simulink model "BandwidthSelector"  (R2019a)
settings: Solver=VariableStepAuto  StartTime=0.0  StopTime=inf  RelTol=1e-3
InitFcn:
  | bandwidthselector_setup;
values from neighbouring files (symbols this model uses):
  f = 256e6    (= 256000000)    [bandwidthselector_setup.m]
undefined symbols (not defined in the file or in its folder): AXI4, designMultirateFIR, Lite, xlfda_numerator
libraries: xbsIndex_r4 x43, dspmlti4 x6, dspswit3 x4, dspsigops x2
(part 1 of 2)
settings Model: Creator=rgb11127  LastModifiedBy=david
settings DataIOCC: ReturnWorkspaceOutputs=off
settings DebuggingCC: PregeneratedLibrarySubsystemCodeDiagnostic=none  ArithmeticOperatorsInVariantConditions=warning
settings SFSimCC: SimUseLocalCustomCode=off
settings RTWCC: RTWUseLocalCustomCode=off

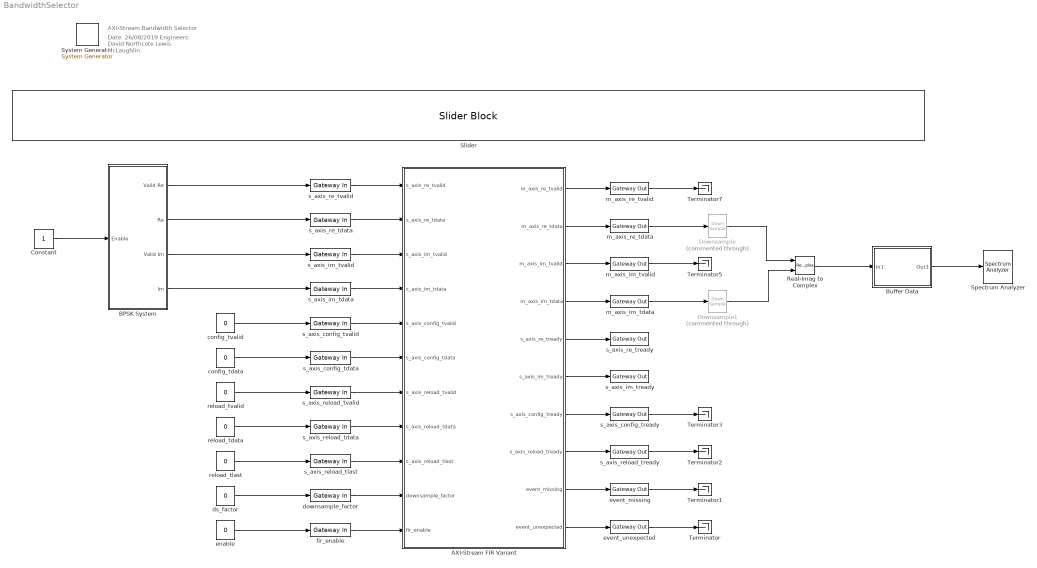
== system BandwidthSelector ==
  note: Date: 26/08/2019
      | Engineers: David Northcote
      | Lewis McLaughlin
  note: AXI-Stream Bandwidth Selector
  " System Generator" : xbsIndex_r4/ System Generator  Tag=genX  xilinxfamily=zynquplusRFSOC  part=xczu28dr  speed=-2-e  package=ffvg1517  synthesis_tool=Vivado  clock_wrapper=Clock Enables  directory=./netlist  proj_type=Vivado  Synth_file=Vivado Synthesis Defaults  Impl_file=Vivado Implementation Defaults  testbench=off  simulink_period=1/f  sysclk_period=(1/f)*1e9  dcm_input_clock_period=10  incr_netlist=off  trim_vbits=Everywhere in SubSystem  dbl_ovrd=According to Block Masks  core_generation=According to Block Masks  run_coregen=off  deprecated_control=off  eval_field=0  block_type=sysgen
  AXI-Stream FIR Variant : Subsystem  AncestorBlock=lib_fir/AXI-Stream FIR Variant  VariantControlMode=Label  Variant=on  VariantControl=Variant1  LabelModeActiveChoice=Variant
  BPSK System : Subsystem
  Buffer Data : Subsystem
  Constant : Constant  SampleTime=-1
  Downsample : DownSample  Commented=through  N=1  RateOptions=Allow multirate processing
  Downsample1 : DownSample  Commented=through  N=1  RateOptions=Allow multirate processing
  Real-Imag to Complex : RealImagToComplex
  Slider : SliderBlock  ScaleMax=128000000  TickInterval=4000000
  Spectrum Analyzer : SpectrumAnalyzer
  Terminator{,1..3,5,7} (6 alike) : Terminator
  config_tdata : Constant  Value=0  OutDataTypeStr=fixdt(0,8,0)  SampleTime=1/f
  config_tvalid : Constant  Value=0  OutDataTypeStr=boolean  SampleTime=1/f
  downsample_factor : xbsIndex_r4/Gateway In  gui_display_data_type=Fixed-point  arith_type=Unsigned  n_bits=32  bin_pt=0  preci_type=Single  exp_width=8  frac_width=24  rows=1  columns=1  quantization=Truncate  overflow=Wrap  period=1/f  UseAsADC=off  ADCChannel='1'  interface=AXI4-Lite  automatic_assignment=on  address_offset=hex2dec('00')  intf_name=''  intf_description=''  default_value=1  timing_constraint=None  locs_specified=off  LOCs={}  io_standard={}  inherit_from_input=off  hdl_port=on  dbl_ovrd=off  block_type=gatewayin
  ds_factor : Constant  Value=0  OutDataTypeStr=uint16  SampleTime=1/f
  enable : Constant  Value=0  OutDataTypeStr=uint32  SampleTime=1/f
  event_missing : xbsIndex_r4/Gateway Out  inherit_from_input=on  hdl_port=on  rows=1  columns=1  UseAsDAC=off  DACChannel='1'  interface=AXI4-Lite  automatic_assignment=on  address_offset=hex2dec('00')  intf_name=''  intf_description=''  timing_constraint=None  locs_specified=off  LOCs={}  io_standard={}  block_type=gatewayout
  event_unexpected : xbsIndex_r4/Gateway Out  inherit_from_input=on  hdl_port=on  rows=1  columns=1  UseAsDAC=off  DACChannel='1'  interface=AXI4-Lite  automatic_assignment=on  address_offset=hex2dec('00')  intf_name=''  intf_description=''  timing_constraint=None  locs_specified=off  LOCs={}  io_standard={}  block_type=gatewayout
  fir_enable : xbsIndex_r4/Gateway In  gui_display_data_type=Fixed-point  arith_type=Unsigned  n_bits=8  bin_pt=0  preci_type=Single  exp_width=8  frac_width=24  rows=1  columns=1  quantization=Truncate  overflow=Saturate  period=1/f  UseAsADC=off  ADCChannel='1'  interface=AXI4-Lite  automatic_assignment=on  address_offset=hex2dec('00')  intf_name=''  intf_description=''  default_value=1  timing_constraint=None  locs_specified=off  LOCs={}  io_standard={}  inherit_from_input=off  hdl_port=on  dbl_ovrd=off  block_type=gatewayin
  m_axis_im_tdata : xbsIndex_r4/Gateway Out  inherit_from_input=on  hdl_port=on  rows=1  columns=1  UseAsDAC=off  DACChannel='1'  interface=None  automatic_assignment=on  address_offset=hex2dec('00')  intf_name=''  intf_description=''  timing_constraint=None  locs_specified=off  LOCs={}  io_standard={}  block_type=gatewayout
  m_axis_im_tvalid : xbsIndex_r4/Gateway Out  inherit_from_input=on  hdl_port=on  rows=1  columns=1  UseAsDAC=off  DACChannel='1'  interface=None  automatic_assignment=on  address_offset=hex2dec('00')  intf_name=''  intf_description=''  timing_constraint=None  locs_specified=off  LOCs={}  io_standard={}  block_type=gatewayout
  m_axis_re_tdata : xbsIndex_r4/Gateway Out  inherit_from_input=on  hdl_port=on  rows=1  columns=1  UseAsDAC=off  DACChannel='1'  interface=None  automatic_assignment=on  address_offset=hex2dec('00')  intf_name=''  intf_description=''  timing_constraint=None  locs_specified=off  LOCs={}  io_standard={}  block_type=gatewayout
  m_axis_re_tvalid : xbsIndex_r4/Gateway Out  inherit_from_input=on  hdl_port=on  rows=1  columns=1  UseAsDAC=off  DACChannel='1'  interface=None  automatic_assignment=on  address_offset=hex2dec('00')  intf_name=''  intf_description=''  timing_constraint=None  locs_specified=off  LOCs={}  io_standard={}  block_type=gatewayout
  reload_tdata : Constant  Value=0  OutDataTypeStr=fixdt(0,12,0)  SampleTime=1/f
  reload_tlast : Constant  Value=0  OutDataTypeStr=boolean  SampleTime=1/f
  reload_tvalid : Constant  Value=0  OutDataTypeStr=boolean  SampleTime=1/f
  s_axis_config_tdata : xbsIndex_r4/Gateway In  gui_display_data_type=Fixed-point  arith_type=Unsigned  n_bits=8  bin_pt=0  preci_type=Single  exp_width=8  frac_width=24  rows=1  columns=1  quantization="Round  (unbiased: +/- Inf)"  overflow=Saturate  period=1/f  UseAsADC=off  ADCChannel='1'  interface=None  automatic_assignment=on  address_offset=hex2dec('00')  intf_name=''  intf_description=''  default_value=0  timing_constraint=None  locs_specified=off  LOCs={}  io_standard={}  inherit_from_input=off  hdl_port=on  dbl_ovrd=off  block_type=gatewayin
  s_axis_config_tready : xbsIndex_r4/Gateway Out  inherit_from_input=on  hdl_port=on  rows=1  columns=1  UseAsDAC=off  DACChannel='1'  interface=None  automatic_assignment=on  address_offset=hex2dec('00')  intf_name=''  intf_description=''  timing_constraint=None  locs_specified=off  LOCs={}  io_standard={}  block_type=gatewayout
  s_axis_config_tvalid : xbsIndex_r4/Gateway In  gui_display_data_type=Boolean  arith_type=Boolean  n_bits=16  bin_pt=14  preci_type=Single  exp_width=8  frac_width=24  rows=1  columns=1  quantization="Round  (unbiased: +/- Inf)"  overflow=Saturate  period=1/f  UseAsADC=off  ADCChannel='1'  interface=None  automatic_assignment=on  address_offset=hex2dec('00')  intf_name=''  intf_description=''  default_value=0  timing_constraint=None  locs_specified=off  LOCs={}  io_standard={}  inherit_from_input=off  hdl_port=on  dbl_ovrd=off  block_type=gatewayin
  s_axis_im_tdata : xbsIndex_r4/Gateway In  gui_display_data_type=Fixed-point  arith_type="Signed  (2's comp)"  n_bits=16  bin_pt=15  preci_type=Single  exp_width=8  frac_width=24  rows=1  columns=1  quantization="Round  (unbiased: +/- Inf)"  overflow=Saturate  period=1/f  UseAsADC=off  ADCChannel='1'  interface=None  automatic_assignment=on  address_offset=hex2dec('00')  intf_name=''  intf_description=''  default_value=0  timing_constraint=None  locs_specified=off  LOCs={}  io_standard={}  inherit_from_input=off  hdl_port=on  dbl_ovrd=off  block_type=gatewayin
  s_axis_im_tready : xbsIndex_r4/Gateway Out  inherit_from_input=on  hdl_port=on  rows=1  columns=1  UseAsDAC=off  DACChannel='1'  interface=None  automatic_assignment=on  address_offset=hex2dec('00')  intf_name=''  intf_description=''  timing_constraint=None  locs_specified=off  LOCs={}  io_standard={}  block_type=gatewayout
  s_axis_im_tvalid : xbsIndex_r4/Gateway In  gui_display_data_type=Boolean  arith_type=Boolean  n_bits=16  bin_pt=14  preci_type=Single  exp_width=8  frac_width=24  rows=1  columns=1  quantization="Round  (unbiased: +/- Inf)"  overflow=Saturate  period=1/f  UseAsADC=off  ADCChannel='1'  interface=None  automatic_assignment=on  address_offset=hex2dec('00')  intf_name=''  intf_description=''  default_value=0  timing_constraint=None  locs_specified=off  LOCs={}  io_standard={}  inherit_from_input=off  hdl_port=on  dbl_ovrd=off  block_type=gatewayin
  s_axis_re_tdata : xbsIndex_r4/Gateway In  gui_display_data_type=Fixed-point  arith_type="Signed  (2's comp)"  n_bits=16  bin_pt=15  preci_type=Single  exp_width=8  frac_width=24  rows=1  columns=1  quantization="Round  (unbiased: +/- Inf)"  overflow=Saturate  period=1/f  UseAsADC=off  ADCChannel='1'  interface=None  automatic_assignment=on  address_offset=hex2dec('00')  intf_name=''  intf_description=''  default_value=0  timing_constraint=None  locs_specified=off  LOCs={}  io_standard={}  inherit_from_input=off  hdl_port=on  dbl_ovrd=off  block_type=gatewayin
  s_axis_re_tready : xbsIndex_r4/Gateway Out  inherit_from_input=on  hdl_port=on  rows=1  columns=1  UseAsDAC=off  DACChannel='1'  interface=None  automatic_assignment=on  address_offset=hex2dec('00')  intf_name=''  intf_description=''  timing_constraint=None  locs_specified=off  LOCs={}  io_standard={}  block_type=gatewayout
  s_axis_re_tvalid : xbsIndex_r4/Gateway In  gui_display_data_type=Boolean  arith_type=Boolean  n_bits=16  bin_pt=14  preci_type=Single  exp_width=8  frac_width=24  rows=1  columns=1  quantization="Round  (unbiased: +/- Inf)"  overflow=Saturate  period=1/f  UseAsADC=off  ADCChannel='1'  interface=None  automatic_assignment=on  address_offset=hex2dec('00')  intf_name=''  intf_description=''  default_value=0  timing_constraint=None  locs_specified=off  LOCs={}  io_standard={}  inherit_from_input=off  hdl_port=on  dbl_ovrd=off  block_type=gatewayin
  s_axis_reload_tdata : xbsIndex_r4/Gateway In  gui_display_data_type=Fixed-point  arith_type=Unsigned  n_bits=16  bin_pt=0  preci_type=Single  exp_width=8  frac_width=24  rows=1  columns=1  quantization="Round  (unbiased: +/- Inf)"  overflow=Saturate  period=1/f  UseAsADC=off  ADCChannel='1'  interface=None  automatic_assignment=on  address_offset=hex2dec('00')  intf_name=''  intf_description=''  default_value=0  timing_constraint=None  locs_specified=off  LOCs={}  io_standard={}  inherit_from_input=off  hdl_port=on  dbl_ovrd=off  block_type=gatewayin
  s_axis_reload_tlast : xbsIndex_r4/Gateway In  gui_display_data_type=Boolean  arith_type=Boolean  n_bits=16  bin_pt=14  preci_type=Single  exp_width=8  frac_width=24  rows=1  columns=1  quantization="Round  (unbiased: +/- Inf)"  overflow=Saturate  period=1/f  UseAsADC=off  ADCChannel='1'  interface=None  automatic_assignment=on  address_offset=hex2dec('00')  intf_name=''  intf_description=''  default_value=0  timing_constraint=None  locs_specified=off  LOCs={}  io_standard={}  inherit_from_input=off  hdl_port=on  dbl_ovrd=off  block_type=gatewayin
  s_axis_reload_tready : xbsIndex_r4/Gateway Out  inherit_from_input=on  hdl_port=on  rows=1  columns=1  UseAsDAC=off  DACChannel='1'  interface=None  automatic_assignment=on  address_offset=hex2dec('00')  intf_name=''  intf_description=''  timing_constraint=None  locs_specified=off  LOCs={}  io_standard={}  block_type=gatewayout
  s_axis_reload_tvalid : xbsIndex_r4/Gateway In  gui_display_data_type=Boolean  arith_type=Boolean  n_bits=16  bin_pt=14  preci_type=Single  exp_width=8  frac_width=24  rows=1  columns=1  quantization="Round  (unbiased: +/- Inf)"  overflow=Saturate  period=1/f  UseAsADC=off  ADCChannel='1'  interface=None  automatic_assignment=on  address_offset=hex2dec('00')  intf_name=''  intf_description=''  default_value=0  timing_constraint=None  locs_specified=off  LOCs={}  io_standard={}  inherit_from_input=off  hdl_port=on  dbl_ovrd=off  block_type=gatewayin
  wires:
  reload_tlast/1 -> s_axis_reload_tlast/1
  reload_tdata/1 -> s_axis_reload_tdata/1
  config_tdata/1 -> s_axis_config_tdata/1
  reload_tvalid/1 -> s_axis_reload_tvalid/1
  config_tvalid/1 -> s_axis_config_tvalid/1
  AXI-Stream FIR Variant/5(s_axis_re_tready) -> s_axis_re_tready/1
  AXI-Stream FIR Variant/6(s_axis_im_tready) -> s_axis_im_tready/1
  AXI-Stream FIR Variant/10(event_unexpected) -> event_unexpected/1
  AXI-Stream FIR Variant/9(event_missing) -> event_missing/1
  AXI-Stream FIR Variant/8(" s_axis_reload_tready") -> s_axis_reload_tready/1
  AXI-Stream FIR Variant/7(" s_axis_config_tready") -> s_axis_config_tready/1
  AXI-Stream FIR Variant/4(" m_axis_im_tdata") -> m_axis_im_tdata/1
  AXI-Stream FIR Variant/3(" m_axis_im_tvalid") -> m_axis_im_tvalid/1
  AXI-Stream FIR Variant/2(" m_axis_re_tdata") -> m_axis_re_tdata/1
  AXI-Stream FIR Variant/1(" m_axis_re_tvalid") -> m_axis_re_tvalid/1
  s_axis_re_tvalid/1 -> AXI-Stream FIR Variant/1("s_axis_re_tvalid ")
  s_axis_im_tvalid/1 -> AXI-Stream FIR Variant/3(s_axis_im_tvalid)
  s_axis_re_tdata/1 -> AXI-Stream FIR Variant/2(s_axis_re_tdata)
  s_axis_im_tdata/1 -> AXI-Stream FIR Variant/4(s_axis_im_tdata)
  s_axis_config_tvalid/1 -> AXI-Stream FIR Variant/5(s_axis_config_tvalid)
  s_axis_reload_tvalid/1 -> AXI-Stream FIR Variant/7(s_axis_reload_tvalid)
  s_axis_reload_tlast/1 -> AXI-Stream FIR Variant/9(s_axis_reload_tlast)
  s_axis_config_tdata/1 -> AXI-Stream FIR Variant/6(s_axis_config_tdata)
  s_axis_reload_tdata/1 -> AXI-Stream FIR Variant/8(s_axis_reload_tdata)
  m_axis_re_tvalid/1 -> Terminator7/1
  m_axis_im_tvalid/1 -> Terminator5/1
  s_axis_config_tready/1 -> Terminator3/1
  s_axis_reload_tready/1 -> Terminator2/1
  event_missing/1 -> Terminator1/1
  event_unexpected/1 -> Terminator/1
  Constant/1 -> BPSK System/1(Enable)
  downsample_factor/1 -> AXI-Stream FIR Variant/10(downsample_factor)
  ds_factor/1 -> downsample_factor/1
  enable/1 -> fir_enable/1
  fir_enable/1 -> AXI-Stream FIR Variant/11(fir_enable)
  Downsample/1 -> Real-Imag to Complex/1
  Downsample1/1 -> Real-Imag to Complex/2
  Real-Imag to Complex/1 -> Buffer Data/1(In1)
  Buffer Data/1(Out1) -> Spectrum Analyzer/1
  m_axis_im_tdata/1 -> Downsample1/1
  m_axis_re_tdata/1 -> Downsample/1
  BPSK System/2(Re) -> s_axis_re_tdata/1
  BPSK System/1(Valid Re) -> s_axis_re_tvalid/1
  BPSK System/3(Valid Im) -> s_axis_im_tvalid/1
  BPSK System/4(Im) -> s_axis_im_tdata/1

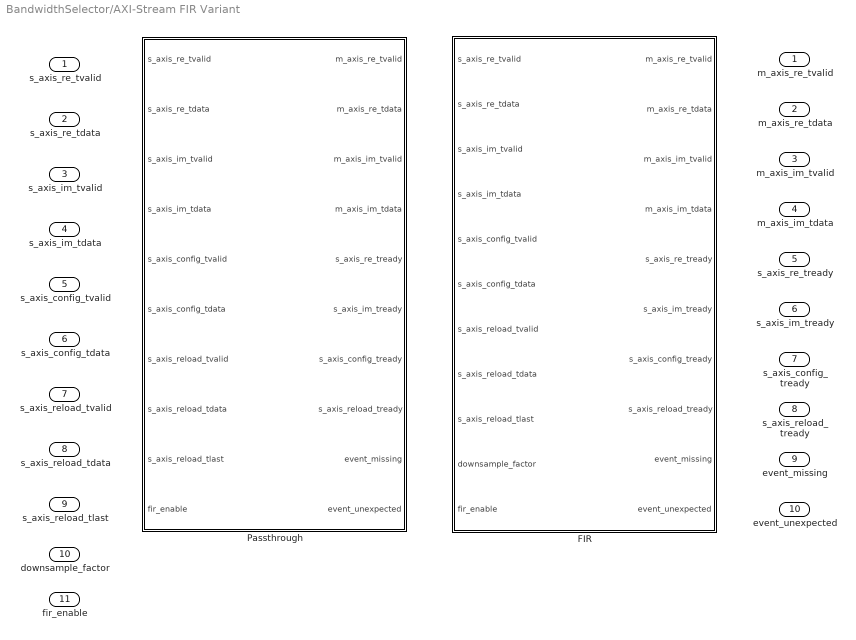
== system BandwidthSelector/AXI-Stream FIR Variant ==
  "s_axis_re_tvalid " : Inport
  s_axis_re_tdata : Inport  Port=2
  s_axis_im_tvalid : Inport  Port=3
  s_axis_im_tdata : Inport  Port=4
  s_axis_config_tvalid : Inport  Port=5
  s_axis_config_tdata : Inport  Port=6
  s_axis_reload_tvalid : Inport  Port=7
  s_axis_reload_tdata : Inport  Port=8
  s_axis_reload_tlast : Inport  Port=9
  downsample_factor : Inport  Port=10
  fir_enable : Inport  Port=11
  FIR : Subsystem  VariantControl=Variant
  Passthrough : Subsystem  VariantControl=Variant1
  " m_axis_re_tvalid" : Outport
  " m_axis_re_tdata" : Outport  Port=2
  " m_axis_im_tvalid" : Outport  Port=3
  " m_axis_im_tdata" : Outport  Port=4
  s_axis_re_tready : Outport  Port=5
  s_axis_im_tready : Outport  Port=6
  " s_axis_config_tready" : Outport  Port=7
  " s_axis_reload_tready" : Outport  Port=8
  event_missing : Outport  Port=9
  event_unexpected : Outport  Port=10

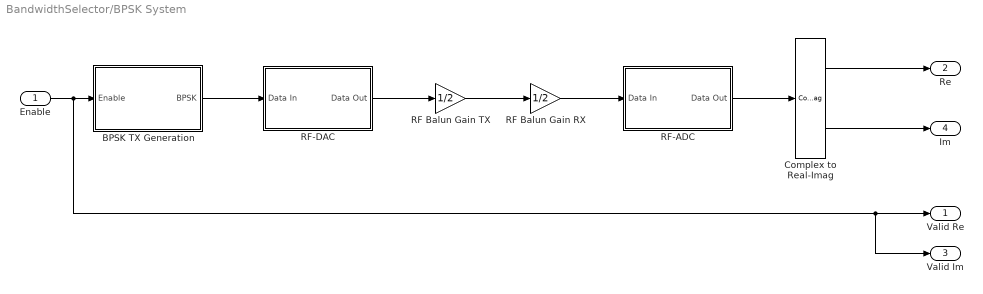
== system BandwidthSelector/BPSK System ==
  Enable : Inport
  BPSK TX Generation : Subsystem
  Complex to Real-Imag : ComplexToRealImag
  RF Balun Gain RX : Gain  Gain=1/2
  RF Balun Gain TX : Gain  Gain=1/2
  RF-ADC : Subsystem  mask{fs_ghz=2.048, decim=8x, ssr=1, mode=Fine, fc=0.064, fph=0, fcoarse=fs/4}
      mask prompts: fs_ghz "Sample Rate (GHz):"; decim "Interpolation Mode:"; ssr "Samples per AXI4-Stream Cycle:"; mode "Mixer Type:"; fc "NCO Frequency (GHz):"; fph "NCO Phase (Rads):"; fcoarse "Frequency:"
      mask init:
      | % Obtain the sample rate in Hz
      | fs = str2double(get_param(gcb, 'fs_ghz'))*1e9;
      | 
      | % Set the mode of the RF-DAC interpolation filter
      | switch get_param(gcb, 'decim')
      |     case '1x'
      |         D = 1;
      |     case '2x'
      |         D = 2;
      |     case '4x'
      |         D = 4;
      |     case '8x'
      |         D = 8;
      |     otherwise
      |         D = 1;
      | end
      | 
      | % Get the AXI-Stream clock for display to user
      | axi_clk = (fs/(str2double(get_param(gcb, 'ssr'))*D))*1e-6;
      | 
      | % Get the block mask object to manipulate settings
      | mo = get_param(gcb, 'MaskObject');
      | 
      | % Update text to display the required AXI-Stream clock
      | tc = mo.getDialogControl('axi_text');
      | tc.Prompt = ['      Required AXI-Stream Clock: ', num2str(axi_clk), ' MHz'];
      | 
      | % Set the RF-DAC Mixer mode
      | switch get_param(gcb, 'mode')
      |     case 'Bypass'
      |         m = 0;
      |     case 'Coarse'
      |         m = 1;
      |     case 'Fine'
      |         m = 2;
      |     otherwise
      |         m = 0;
      | end
      | 
      | % Set the RF-DAC Coarse Mixer mode
      | switch get_param(gcb, 'fcoarse')
      |     case 'fs/2'
      |         mc = 0;
      |     case 'fs/4'
      |         mc = 1;
      |     case '-fs/4'
      |         mc = 2;
      |     otherwise
      |         mc = 0;
      | end
      | 
      | % Set other blocks
      | set_param([gcb, '/Decimation Filter'], 'decim', get_param(gcb, 'decim'));
      mask Callback fs_ghz:
      | % Obtain the sample rate in Hz
      | fs = str2double(get_param(gcb, 'fs_ghz'))*1e9;
      | 
      | % Set the mode of the RF-DAC interpolation filter
      | switch get_param(gcb, 'decim')
      |     case '1x'
      |         D = 1;
      |     case '2x'
      |         D = 2;
      |     case '4x'
      |         D = 4;
      |     case '8x'
      |         D = 8;
      |     otherwise
      |         D = 1;
      | end
      | 
      | % Get the AXI-Stream clock for display to user
      | axi_clk = (fs/(str2double(get_param(gcb, 'ssr'))*D))*1e-6;
      | 
      | % Get the block mask object to manipulate settings
      | mo = get_param(gcb, 'MaskObject');
      | 
      | % Update text to display the required AXI-Stream clock
      | tc = mo.getDialogControl('axi_text');
      | tc.Prompt = ['      Required AXI-Stream Clock: ', num2str(axi_clk), ' MHz'];
      mask TypeOptions decim: 1x | 2x | 4x | 8x
      mask Callback decim:
      | % Obtain the sample rate in Hz
      | fs = str2double(get_param(gcb, 'fs_ghz'))*1e9;
      | 
      | % Set the mode of the RF-DAC interpolation filter
      | switch get_param(gcb, 'decim')
      |     case '1x'
      |         D = 1;
      |     case '2x'
      |         D = 2;
      |     case '4x'
      |         D = 4;
      |     case '8x'
      |         D = 8;
      |     otherwise
      |         D = 1;
      | end
      | 
      | % Get the AXI-Stream clock for display to user
      | axi_clk = (fs/(str2double(get_param(gcb, 'ssr'))*D))*1e-6;
      | 
      | % Get the block mask object to manipulate settings
      | mo = get_param(gcb, 'MaskObject');
      | 
      | % Update text to display the required AXI-Stream clock
      | tc = mo.getDialogControl('axi_text');
      | tc.Prompt = ['      Required AXI-Stream Clock: ', num2str(axi_clk), ' MHz'];
      mask TypeOptions ssr: 1 | 2 | 3 | 4 | 5 | 6 | 7 | 8 | 9 | 10 | 11 | 12 | 13 | 14 | 15 | 16
      mask Callback ssr:
      | % Obtain the sample rate in Hz
      | fs = str2double(get_param(gcb, 'fs_ghz'))*1e9;
      | 
      | % Set the mode of the RF-DAC interpolation filter
      | switch get_param(gcb, 'decim')
      |     case '1x'
      |         D = 1;
      |     case '2x'
      |         D = 2;
      |     case '4x'
      |         D = 4;
      |     case '8x'
      |         D = 8;
      |     otherwise
      |         D = 1;
      | end
      | 
      | % Get the AXI-Stream clock for display to user
      | axi_clk = (fs/(str2double(get_param(gcb, 'ssr'))*D))*1e-6;
      | 
      | % Get the block mask object to manipulate settings
      | mo = get_param(gcb, 'MaskObject');
      | 
      | % Update text to display the required AXI-Stream clock
      | tc = mo.getDialogControl('axi_text');
      | tc.Prompt = ['      Required AXI-Stream Clock: ', num2str(axi_clk), ' MHz'];
      mask TypeOptions mode: Coarse | Fine
      mask Callback mode:
      | % Get the block mask object to manipulate settings
      | mo = get_param(gcb, 'MaskObject');
      | 
      | % Hide group depending on Mixer mode choice
      | switch get_param(gcb, 'mode')
      |     case 'Bypass'
      |         mo.getDialogControl('coarse_group').Visible='off';
      |         mo.getDialogControl('mixer_group').Visible='off';
      |     case 'Coarse'
      |         mo.getDialogControl('coarse_group').Visible='on';
      |         mo.getDialogControl('mixer_group').Visible='off';
      |     case 'Fine'
      |         mo.getDialogControl('coarse_group').Visible='off';
      |         mo.getDialogControl('mixer_group').Visible='on';
      |     otherwise
      |         mo.getDialogControl('coarse_group').Visible='off';
      |         mo.getDialogControl('mixer_group').Visible='off';
      | end
      mask TypeOptions fcoarse: fs/2 | fs/4 | -fs/4
      mask DialogControl DescGroupVar Prompt: RF-DAC
      mask DialogControl DescTextVar Prompt: This block simulates one RF-ADC channel.
      mask DialogControl main_group Prompt: Data Settings
      mask DialogControl axi_text Prompt: Required AXI-Stream Clock: 256 MHz
      mask DialogControl Container5 Prompt: Mixer Settings
  RF-DAC : Subsystem  mask{fs_ghz=2.048, interp=8x, ssr=1, mode=Fine, fc=0.032, fph=0, fcoarse=fs/4}
      mask prompts: fs_ghz "Sample Rate (GHz):"; interp "Interpolation Mode:"; ssr "Samples per AXI4-Stream Cycle:"; mode "Mixer Type:"; fc "NCO Frequency (GHz):"; fph "NCO Phase (Rads):"; fcoarse "Frequency:"
      mask init:
      | % Obtain the sample rate in Hz
      | fs = str2double(get_param(gcb, 'fs_ghz'))*1e9;
      | 
      | % Set the mode of the RF-DAC interpolation filter
      | switch get_param(gcb, 'interp')
      |     case '1x'
      |         L = 1;
      |     case '2x'
      |         L = 2;
      |     case '4x'
      |         L = 4;
      |     case '8x'
      |         L = 8;
      |     otherwise
      |         L = 1;
      | end
      | 
      | % Get the AXI-Stream clock for display to user
      | axi_clk = (fs/(str2double(get_param(gcb, 'ssr'))*L))*1e-6;
      | 
      | % Get the block mask object to manipulate settings
      | mo = get_param(gcb, 'MaskObject');
      | 
      | % Update text to display the required AXI-Stream clock
      | tc = mo.getDialogControl('axi_text');
      | tc.Prompt = ['      Required AXI-Stream Clock: ', num2str(axi_clk), ' MHz'];
      | 
      | % Set the RF-DAC Mixer mode
      | switch get_param(gcb, 'mode')
      |     case 'Bypass'
      |         m = 0;
      |     case 'Coarse'
      |         m = 1;
      |     case 'Fine'
      |         m = 2;
      |     otherwise
      |         m = 0;
      | end
      | 
      | % Set the RF-DAC Coarse Mixer mode
      | switch get_param(gcb, 'fcoarse')
      |     case 'fs/2'
      |         mc = 0;
      |     case 'fs/4'
      |         mc = 1;
      |     case '-fs/4'
      |         mc = 2;
      |     otherwise
      |         mc = 0;
      | end
      | 
      | % Set other blocks
      | set_param([gcb, '/Interpolation Filter'], 'interp', get_param(gcb, 'interp'));
      mask Callback fs_ghz:
      | % Obtain the sample rate in Hz
      | fs = str2double(get_param(gcb, 'fs_ghz'))*1e9;
      | 
      | % Set the mode of the RF-DAC interpolation filter
      | switch get_param(gcb, 'interp')
      |     case '1x'
      |         L = 1;
      |     case '2x'
      |         L = 2;
      |     case '4x'
      |         L = 4;
      |     case '8x'
      |         L = 8;
      |     otherwise
      |         L = 1;
      | end
      | 
      | % Get the AXI-Stream clock for display to user
      | axi_clk = (fs/(str2double(get_param(gcb, 'ssr'))*L))*1e-6;
      | 
      | % Get the block mask object to manipulate settings
      | mo = get_param(gcb, 'MaskObject');
      | 
      | % Update text to display the required AXI-Stream clock
      | tc = mo.getDialogControl('axi_text');
      | tc.Prompt = ['      Required AXI-Stream Clock: ', num2str(axi_clk), ' MHz'];
      mask TypeOptions interp: 1x | 2x | 4x | 8x
      mask Callback interp:
      | % Obtain the sample rate in Hz
      | fs = str2double(get_param(gcb, 'fs_ghz'))*1e9;
      | 
      | % Set the mode of the RF-DAC interpolation filter
      | switch get_param(gcb, 'interp')
      |     case '1x'
      |         L = 1;
      |     case '2x'
      |         L = 2;
      |     case '4x'
      |         L = 4;
      |     case '8x'
      |         L = 8;
      |     otherwise
      |         L = 1;
      | end
      | 
      | % Get the AXI-Stream clock for display to user
      | axi_clk = (fs/(str2double(get_param(gcb, 'ssr'))*L))*1e-6;
      | 
      | % Get the block mask object to manipulate settings
      | mo = get_param(gcb, 'MaskObject');
      | 
      | % Update text to display the required AXI-Stream clock
      | tc = mo.getDialogControl('axi_text');
      | tc.Prompt = ['      Required AXI-Stream Clock: ', num2str(axi_clk), ' MHz'];
      mask TypeOptions ssr: 1 | 2 | 3 | 4 | 5 | 6 | 7 | 8 | 9 | 10 | 11 | 12 | 13 | 14 | 15 | 16
      mask Callback ssr:
      | % Obtain the sample rate in Hz
      | fs = str2double(get_param(gcb, 'fs_ghz'))*1e9;
      | 
      | % Set the mode of the RF-DAC interpolation filter
      | switch get_param(gcb, 'interp')
      |     case '1x'
      |         L = 1;
      |     case '2x'
      |         L = 2;
      |     case '4x'
      |         L = 4;
      |     case '8x'
      |         L = 8;
      |     otherwise
      |         L = 1;
      | end
      | 
      | % Get the AXI-Stream clock for display to user
      | axi_clk = (fs/(str2double(get_param(gcb, 'ssr'))*L))*1e-6;
      | 
      | % Get the block mask object to manipulate settings
      | mo = get_param(gcb, 'MaskObject');
      | 
      | % Update text to display the required AXI-Stream clock
      | tc = mo.getDialogControl('axi_text');
      | tc.Prompt = ['      Required AXI-Stream Clock: ', num2str(axi_clk), ' MHz'];
      mask TypeOptions mode: Coarse | Fine
      mask Callback mode:
      | % Get the block mask object to manipulate settings
      | mo = get_param(gcb, 'MaskObject');
      | 
      | % Hide group depending on Mixer mode choice
      | switch get_param(gcb, 'mode')
      |     case 'Bypass'
      |         mo.getDialogControl('coarse_group').Visible='off';
      |         mo.getDialogControl('mixer_group').Visible='off';
      |     case 'Coarse'
      |         mo.getDialogControl('coarse_group').Visible='on';
      |         mo.getDialogControl('mixer_group').Visible='off';
      |     case 'Fine'
      |         mo.getDialogControl('coarse_group').Visible='off';
      |         mo.getDialogControl('mixer_group').Visible='on';
      |     otherwise
      |         mo.getDialogControl('coarse_group').Visible='off';
      |         mo.getDialogControl('mixer_group').Visible='off';
      | end
      mask TypeOptions fcoarse: fs/2 | fs/4 | -fs/4
      mask DialogControl DescGroupVar Prompt: RF-DAC
      mask DialogControl DescTextVar Prompt: This block simulates one RF-DAC channel.
      mask DialogControl main_group Prompt: Data Settings
      mask DialogControl axi_text Prompt: Required AXI-Stream Clock: 256 MHz
      mask DialogControl Container5 Prompt: Mixer Settings
  Valid Re : Outport
  Re : Outport  Port=2
  Valid Im : Outport  Port=3
  Im : Outport  Port=4
  wires:
  RF-ADC/1(Data Out) -> Complex to Real-Imag/1
  BPSK TX Generation/1(BPSK) -> RF-DAC/1(Data In)
  Enable/1 -> Valid Im/1, Valid Re/1, BPSK TX Generation/1(Enable)
  Complex to Real-Imag/1 -> Re/1
  Complex to Real-Imag/2 -> Im/1
  RF-DAC/1(Data Out) -> RF Balun Gain TX/1
  RF Balun Gain TX/1 -> RF Balun Gain RX/1
  RF Balun Gain RX/1 -> RF-ADC/1(Data In)

== system BandwidthSelector/Buffer Data ==
  In1 : Inport
  Buffer : Buffer  N=2048  OutputFrames=off
  Out1 : Outport
  wires:
  In1/1 -> Buffer/1
  Buffer/1 -> Out1/1

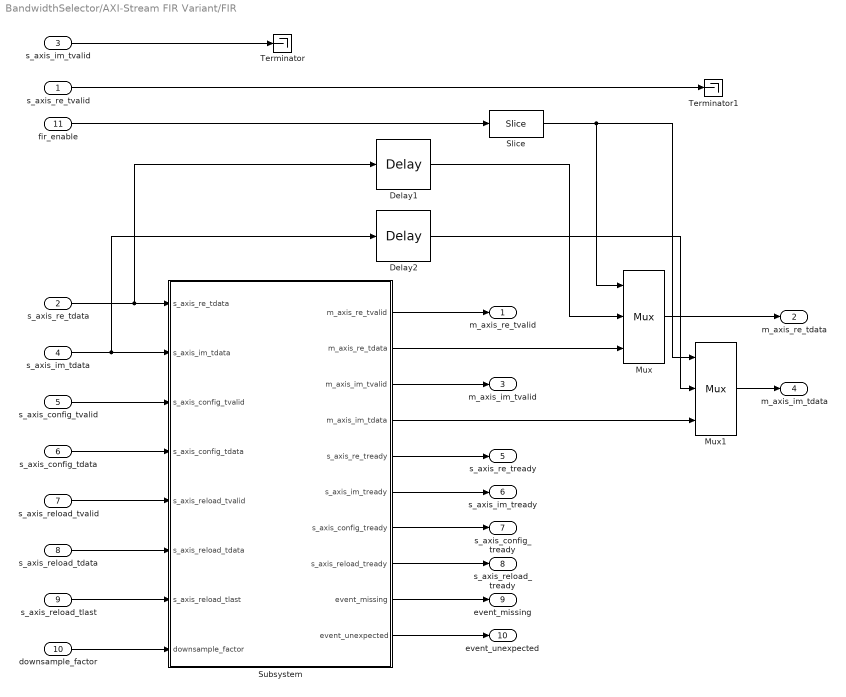
== system BandwidthSelector/AXI-Stream FIR Variant/FIR ==
  "s_axis_re_tvalid " : Inport
  s_axis_re_tdata : Inport  Port=2
  s_axis_im_tvalid : Inport  Port=3
  s_axis_im_tdata : Inport  Port=4
  s_axis_config_tvalid : Inport  Port=5
  s_axis_config_tdata : Inport  Port=6
  s_axis_reload_tvalid : Inport  Port=7
  s_axis_reload_tdata : Inport  Port=8
  s_axis_reload_tlast : Inport  Port=9
  downsample_factor : Inport  Port=10
  fir_enable : Inport  Port=11
  Delay1 : xbsIndex_r4/Delay  rst=off  infoeditControl=Selection of Reset will increase slice count due to use of real FFs and instead of SRLs  en=off  latency=136  reg_retiming=off  dbl_ovrd=off  block_type=delay
  Delay2 : xbsIndex_r4/Delay  rst=off  infoeditControl=Selection of Reset will increase slice count due to use of real FFs and instead of SRLs  en=off  latency=136  reg_retiming=off  dbl_ovrd=off  block_type=delay
  Mux : xbsIndex_r4/Mux  inputs=2  en=off  latency=0  precision=Full  arith_type=Unsigned  n_bits=16  bin_pt=14  quantization=Truncate  overflow=Wrap  dbl_ovrd=off  block_type=mux
  Mux1 : xbsIndex_r4/Mux  inputs=2  en=off  latency=0  precision=Full  arith_type=Unsigned  n_bits=16  bin_pt=14  quantization=Truncate  overflow=Wrap  dbl_ovrd=off  block_type=mux
  Slice : xbsIndex_r4/Slice  nbits=1  boolean_output=off  mode=Two Bit Locations  bit1=0  base1=LSB of Input  bit0=0  base0=LSB of Input  dbl_ovrd=off  block_type=slice
  Subsystem : Subsystem
  Terminator : Terminator
  Terminator1 : Terminator
  " m_axis_re_tvalid" : Outport
  " m_axis_re_tdata" : Outport  Port=2
  " m_axis_im_tvalid" : Outport  Port=3
  " m_axis_im_tdata" : Outport  Port=4
  " s_axis_re_tready" : Outport  Port=5
  " s_axis_im_tready" : Outport  Port=6
  " s_axis_config_tready" : Outport  Port=7
  " s_axis_reload_tready" : Outport  Port=8
  event_missing : Outport  Port=9
  event_unexpected : Outport  Port=10
  wires:
  downsample_factor/1 -> Subsystem/8(downsample_factor)
  Subsystem/10(event_unexpected) -> event_unexpected/1
  Subsystem/9(event_missing) -> event_missing/1
  Subsystem/8(" s_axis_reload_tready") -> " s_axis_reload_tready"/1
  Subsystem/7(" s_axis_config_tready") -> " s_axis_config_tready"/1
  Subsystem/6(" s_axis_im_tready") -> " s_axis_im_tready"/1
  Subsystem/5(" s_axis_re_tready") -> " s_axis_re_tready"/1
  Subsystem/3(" m_axis_im_tvalid") -> " m_axis_im_tvalid"/1
  Subsystem/1(" m_axis_re_tvalid") -> " m_axis_re_tvalid"/1
  s_axis_reload_tlast/1 -> Subsystem/7(s_axis_reload_tlast)
  s_axis_reload_tdata/1 -> Subsystem/6(s_axis_reload_tdata)
  s_axis_reload_tvalid/1 -> Subsystem/5(s_axis_reload_tvalid)
  s_axis_config_tdata/1 -> Subsystem/4(s_axis_config_tdata)
  s_axis_config_tvalid/1 -> Subsystem/3(s_axis_config_tvalid)
  s_axis_re_tdata/1 -> Delay1/1, Subsystem/1(s_axis_re_tdata)
  s_axis_im_tvalid/1 -> Terminator/1
  Subsystem/2(" m_axis_re_tdata") -> Mux/3
  Mux/1 -> " m_axis_re_tdata"/1
  Subsystem/4(" m_axis_im_tdata") -> Mux1/3
  Mux1/1 -> " m_axis_im_tdata"/1
  Delay2/1 -> Mux1/2
  Delay1/1 -> Mux/2
  s_axis_im_tdata/1 -> Delay2/1, Subsystem/2(s_axis_im_tdata)
  fir_enable/1 -> Slice/1
  Slice/1 -> Mux1/1, Mux/1
  "s_axis_re_tvalid "/1 -> Terminator1/1

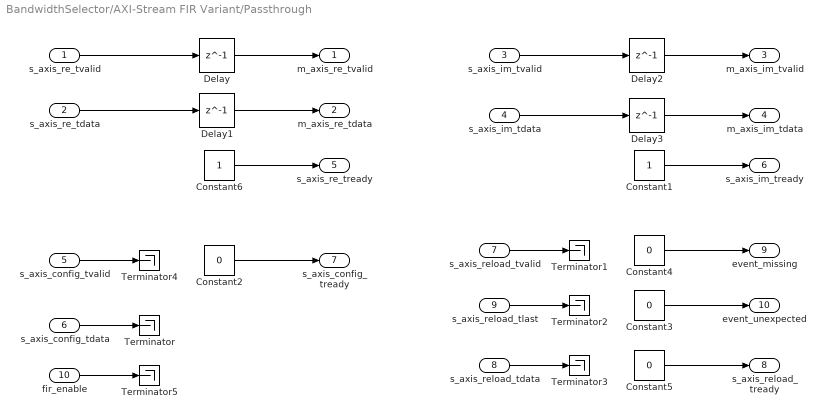
== system BandwidthSelector/AXI-Stream FIR Variant/Passthrough ==
  "s_axis_re_tvalid " : Inport
  s_axis_re_tdata : Inport  Port=2
  s_axis_im_tvalid : Inport  Port=3
  s_axis_im_tdata : Inport  Port=4
  s_axis_config_tvalid : Inport  Port=5
  s_axis_config_tdata : Inport  Port=6
  s_axis_reload_tvalid : Inport  Port=7
  s_axis_reload_tdata : Inport  Port=8
  s_axis_reload_tlast : Inport  Port=9
  fir_enable : Inport  Port=10
  Constant1 : Constant  OutDataTypeStr=boolean  SampleTime=1/f
  Constant{2..5} (4 alike) : Constant  Value=0  OutDataTypeStr=boolean  SampleTime=1/f
  Constant6 : Constant  OutDataTypeStr=boolean  SampleTime=1/f
  Delay{,1..3} (4 alike) : Delay  DelayLength=1
  Terminator{,1..5} (6 alike) : Terminator
  " m_axis_re_tvalid" : Outport
  " m_axis_re_tdata" : Outport  Port=2
  " m_axis_im_tvalid" : Outport  Port=3
  " m_axis_im_tdata" : Outport  Port=4
  " s_axis_re_tready" : Outport  Port=5
  " s_axis_im_tready" : Outport  Port=6
  " s_axis_config_tready" : Outport  Port=7
  " s_axis_reload_tready" : Outport  Port=8
  event_missing : Outport  Port=9
  event_unexpected : Outport  Port=10
  wires:
  Constant5/1 -> " s_axis_reload_tready"/1
  s_axis_config_tdata/1 -> Terminator/1
  s_axis_reload_tlast/1 -> Terminator2/1
  Constant4/1 -> event_missing/1
  s_axis_re_tdata/1 -> Delay1/1
  s_axis_reload_tvalid/1 -> Terminator1/1
  Constant3/1 -> event_unexpected/1
  s_axis_reload_tdata/1 -> Terminator3/1
  Constant1/1 -> " s_axis_im_tready"/1
  Constant2/1 -> " s_axis_config_tready"/1
  s_axis_config_tvalid/1 -> Terminator4/1
  "s_axis_re_tvalid "/1 -> Delay/1
  Constant6/1 -> " s_axis_re_tready"/1
  s_axis_im_tvalid/1 -> Delay2/1
  s_axis_im_tdata/1 -> Delay3/1
  fir_enable/1 -> Terminator5/1
  Delay1/1 -> " m_axis_re_tdata"/1
  Delay/1 -> " m_axis_re_tvalid"/1
  Delay2/1 -> " m_axis_im_tvalid"/1
  Delay3/1 -> " m_axis_im_tdata"/1

== system BandwidthSelector/BPSK System/BPSK TX Generation ==
  Enable : Inport
  Constant : Constant  OutDataTypeStr=fixdt(1,16,15)  SampleTime=-1
  Constant1 : Constant  Value=0  OutDataTypeStr=fixdt(1,16,15)  SampleTime=-1
  Multiport Switch : MultiPortSwitch  DataPortOrder=Zero-based contiguous  Inputs=2  zeroidx=on
  Real-Imag to Complex : RealImagToComplex
  BPSK : Outport
  wires:
  Constant/1 -> Multiport Switch/3
  Enable/1 -> Multiport Switch/1
  Constant1/1 -> Multiport Switch/2
  Multiport Switch/1 -> Real-Imag to Complex/2, Real-Imag to Complex/1
  Real-Imag to Complex/1 -> BPSK/1

== system BandwidthSelector/BPSK System/RF-ADC ==
  Data In : Inport
  Decimation Filter : Subsystem  mask{decim=8x}
      mask prompts: decim "Decimation Factor:"
      mask init:
      | fir0 = dsp.FIRDecimator('DecimationFactor', 2,...
      |                            'CoefficientsDataType', 'Custom',...
      |                            'CustomCoefficientsDataType', numerictype([], 16, 15),...
      |                            'FullPrecisionOverride', false,...
      |                            'OutputDataType', 'Custom',...
      |                            'CustomOutputDataType', numerictype([], 16, 15),...
      |                            'Numerator', [-6, 0 54, 0, -254, 0, 1230, 2048, 1230, 0, -254, 0, 54, 0, -6]/(2048*2));
      | fir1 = dsp.FIRDecimator('DecimationFactor', 2,...
      |                            'CoefficientsDataType', 'Custom',...
      |                            'CustomCoefficientsDataType', numerictype([], 16, 15),...
      |                            'FullPrecisionOverride', false,...
      |                            'OutputDataType', 'Custom',...
      |                            'CustomOutputDataType', numerictype([], 16, 15),...
      |                            'Numerator', [-12, 0, 84, 0, -337, 0, 1008, 0, -2693, 0, 10142, 16384, 10142, 0, -2693, 0, 1008, 0, -337, 0, 84, 0 ,-12]/(16384*2));
      | fir2 = dsp.FIRDecimator('DecimationFactor', 2,...
      |                            'CoefficientsDataType', 'Custom',...
      |                            'CustomCoefficientsDataType', numerictype([], 16, 15),...
      |                            'FullPrecisionOverride', false,...
      |                            'OutputDataType', 'Custom',...
      |                            'CustomOutputDataType', numerictype([], 16, 15),...
      |                            'Numerator', [5, 0, -17, 0, 44, 0, -96, 0, 187, 0, -335, 0, 565, 0, -906, 0, 1401, 0, -2112, 0, 3145, 0, -4723, 0, 7415, 0, -13331, 0, 41526, 65536, 41526, 0, -13331, 0, 7415, 0, -4723, 0, 3145, 0, -2112, 0, 1401, 0, -906, 0, 565, 0, -335, 0, 187, 0, -96, 0, 44, 0, -17, 0, 5]/(65536));
      | switch get_param(gcb, 'decim')
      |     case '1x'
      |         if ~strcmp(get_param([gcb, '/FIR 0'], 'Commented'), 'through')
      |             set_param([gcb, '/FIR 0'],'Commented','through');
      |         end
      |         
      |         if ~strcmp(get_param([gcb, '/FIR 1'], 'Commented'), 'through')
      |             set_param([gcb, '/FIR 1'],'Commented','through');
      |         end
      |         
      |         if ~strcmp(get_param([gcb, '/FIR 2'], 'Commented'), 'through')
      |             set_param([gcb, '/FIR 2'],'Commented','through');
      |         end
      |             
      |     case '2x'
      |         if ~strcmp(get_param([gcb, '/FIR 0'], 'Commented'), 'through')
      |             set_param([gcb, '/FIR 0'],'Commented','through');
      |         end
      |         
      |         if ~strcmp(get_param([gcb, '/FIR 1'], 'Commented'), 'through')
      |             set_param([gcb, '/FIR 1'],'Commented','through');
      |         end
      |         
      |         if ~strcmp(get_param([gcb, '/FIR 2'], 'Commented'), 'off')
      |             set_param([gcb, '/FIR 2'],'Commented','off');
      |         end
      | 
      |     case '4x'
      |         if ~strcmp(get_param([gcb, '/FIR 0'], 'Commented'), 'through')
      |             set_param([gcb, '/FIR 0'],'Commented','through');
      |         end
      |         
      |         if ~strcmp(get_param([gcb, '/FIR 1'], 'Commented'), 'off')
      |             set_param([gcb, '/FIR 1'],'Commented','off');
      |         end
      |         
      |         if ~strcmp(get_param([gcb, '/FIR 2'], 'Commented'), 'off')
      |             set_param([gcb, '/FIR 2'],'Commented','off');
      |         end
      |         
      |     case '8x'
      |         if ~strcmp(get_param([gcb, '/FIR 0'], 'Commented'), 'off')
      |             set_param([gcb, '/FIR 0'],'Commented','off');
      |         end
      |         
      |         if ~strcmp(get_param([gcb, '/FIR 1'], 'Commented'), 'off')
      |             set_param([gcb, '/FIR 1'],'Commented','off');
      |         end
      |         
      |         if ~strcmp(get_param([gcb, '/FIR 2'], 'Commented'), 'off')
      |             set_param([gcb, '/FIR 2'],'Commented','off');
      |         end
      | 
      | end
      mask TypeOptions decim: 1x | 2x | 4x | 8x
      mask DialogControl DescGroupVar Prompt: RF-DAC Interpolation Filter
      mask DialogControl DescTextVar Prompt: This block simulates the RF-DAC interpolation stage using the same coefficients stored in the interpolation filters.
      mask DialogControl ParameterGroupVar Prompt: Main
  NCO and Mixer : Subsystem
  RF-ADC : Subsystem
  Data Out : Outport
  wires:
  NCO and Mixer/1(Data Out) -> Decimation Filter/1(Data In)
  RF-ADC/1(Data Out) -> NCO and Mixer/1(Data In)
  Data In/1 -> RF-ADC/1(Data In)
  Decimation Filter/1(Data Out) -> Data Out/1

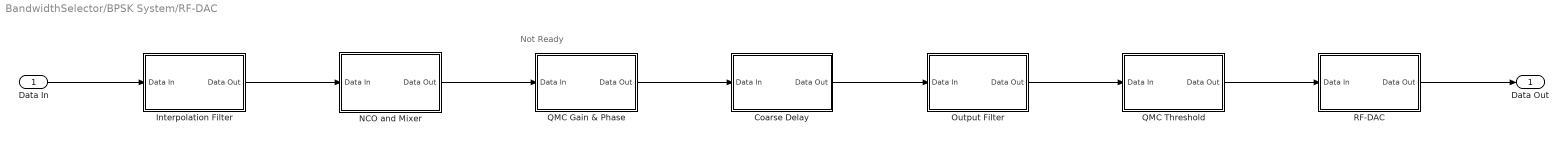
== system BandwidthSelector/BPSK System/RF-DAC ==
  note: Not Ready
  Data In : Inport
  Coarse Delay : Subsystem
  Interpolation Filter : Subsystem  mask{interp=8x}
      mask prompts: interp "Interpolation Factor:"
      mask init:
      | fir0 = dsp.FIRInterpolator('InterpolationFactor', 2,...
      |                            'CoefficientsDataType', 'Custom',...
      |                            'CustomCoefficientsDataType', numerictype([], 16, 15),...
      |                            'FullPrecisionOverride', false,...
      |                            'OutputDataType', 'Custom',...
      |                            'CustomOutputDataType', numerictype([], 16, 15),...
      |                            'Numerator', [-6, 0 54, 0, -254, 0, 1230, 2048, 1230, 0, -254, 0, 54, 0, -6]/(2048));
      | fir1 = dsp.FIRInterpolator('InterpolationFactor', 2,...
      |                            'CoefficientsDataType', 'Custom',...
      |                            'CustomCoefficientsDataType', numerictype([], 16, 15),...
      |                            'FullPrecisionOverride', false,...
      |                            'OutputDataType', 'Custom',...
      |                            'CustomOutputDataType', numerictype([], 16, 15),...
      |                            'Numerator', [-12, 0, 84, 0, -337, 0, 1008, 0, -2693, 0, 10142, 16384, 10142, 0, -2693, 0, 1008, 0, -337, 0, 84, 0 ,-12]/(16384));
      | fir2 = dsp.FIRInterpolator('InterpolationFactor', 2,...
      |                            'CoefficientsDataType', 'Custom',...
      |                            'CustomCoefficientsDataType', numerictype([], 16, 15),...
      |                            'FullPrecisionOverride', false,...
      |                            'OutputDataType', 'Custom',...
      |                            'CustomOutputDataType', numerictype([], 16, 15),...
      |                            'Numerator', [5, 0, -17, 0, 44, 0, -96, 0, 187, 0, -335, 0, 565, 0, -906, 0, 1401, 0, -2112, 0, 3145, 0, -4723, 0, 7415, 0, -13331, 0, 41526, 65536, 41526, 0, -13331, 0, 7415, 0, -4723, 0, 3145, 0, -2112, 0, 1401, 0, -906, 0, 565, 0, -335, 0, 187, 0, -96, 0, 44, 0, -17, 0, 5]/(65536));
      | switch get_param(gcb, 'interp')
      |     case '1x'
      |         if ~strcmp(get_param([gcb, '/FIR 0'], 'Commented'), 'through')
      |             set_param([gcb, '/FIR 0'],'Commented','through');
      |         end
      |         
      |         if ~strcmp(get_param([gcb, '/FIR 1'], 'Commented'), 'through')
      |             set_param([gcb, '/FIR 1'],'Commented','through');
      |         end
      |         
      |         if ~strcmp(get_param([gcb, '/FIR 2'], 'Commented'), 'through')
      |             set_param([gcb, '/FIR 2'],'Commented','through');
      |         end
      |             
      |     case '2x'
      |         if ~strcmp(get_param([gcb, '/FIR 0'], 'Commented'), 'through')
      |             set_param([gcb, '/FIR 0'],'Commented','through');
      |         end
      |         
      |         if ~strcmp(get_param([gcb, '/FIR 1'], 'Commented'), 'through')
      |             set_param([gcb, '/FIR 1'],'Commented','through');
      |         end
      |         
      |         if ~strcmp(get_param([gcb, '/FIR 2'], 'Commented'), 'off')
      |             set_param([gcb, '/FIR 2'],'Commented','off');
      |         end
      | 
      |     case '4x'
      |         if ~strcmp(get_param([gcb, '/FIR 0'], 'Commented'), 'through')
      |             set_param([gcb, '/FIR 0'],'Commented','through');
      |         end
      |         
      |         if ~strcmp(get_param([gcb, '/FIR 1'], 'Commented'), 'off')
      |             set_param([gcb, '/FIR 1'],'Commented','off');
      |         end
      |         
      |         if ~strcmp(get_param([gcb, '/FIR 2'], 'Commented'), 'off')
      |             set_param([gcb, '/FIR 2'],'Commented','off');
      |         end
      |         
      |     case '8x'
      |         if ~strcmp(get_param([gcb, '/FIR 0'], 'Commented'), 'off')
      |             set_param([gcb, '/FIR 0'],'Commented','off');
      |         end
      |         
      |         if ~strcmp(get_param([gcb, '/FIR 1'], 'Commented'), 'off')
      |             set_param([gcb, '/FIR 1'],'Commented','off');
      |         end
      |         
      |         if ~strcmp(get_param([gcb, '/FIR 2'], 'Commented'), 'off')
      |             set_param([gcb, '/FIR 2'],'Commented','off');
      |         end
      | 
      | end
      mask TypeOptions interp: 1x | 2x | 4x | 8x
      mask DialogControl DescGroupVar Prompt: RF-DAC Interpolation Filter
      mask DialogControl DescTextVar Prompt: This block simulates the RF-DAC interpolation stage using the same coefficients stored in the interpolation filters.
      mask DialogControl ParameterGroupVar Prompt: Main
  NCO and Mixer : Subsystem
  Output Filter : Subsystem
  QMC Gain & Phase : Subsystem
  QMC Threshold : Subsystem
  RF-DAC : Subsystem
  Data Out : Outport
  wires:
  RF-DAC/1(Data Out) -> Data Out/1
  QMC Threshold/1(Data Out) -> RF-DAC/1(Data In)
  Output Filter/1(Data Out) -> QMC Threshold/1(Data In)
  Coarse Delay/1(Data Out) -> Output Filter/1(Data In)
  QMC Gain & Phase/1(Data Out) -> Coarse Delay/1(Data In)
  Data In/1 -> Interpolation Filter/1(Data In)
  NCO and Mixer/1(Data Out) -> QMC Gain & Phase/1(Data In)
  Interpolation Filter/1(Data Out) -> NCO and Mixer/1(Data In)
